simulink model "sim_generate_data"  (R2020b)
settings: Solver=FixedStepAuto  StartTime=0.0  StopTime=tsim  FixedStep=dt  RelTol=1e-3
undefined symbols (not defined in the file): A, B, C, dt, Fdiff_lin, Fsum_lin, K, Lobs, NOISE, noise_bound_data, t_disturb, u_disturb, x0
settings Model: Creator=Fabian  LastModifiedBy=Fabian

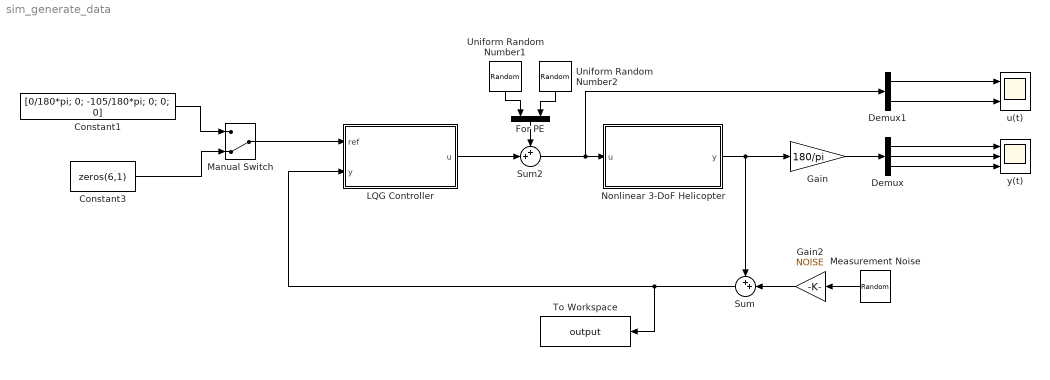
== system sim_generate_data ==
  Constant1 : Constant  Value=[0/180*pi; 0; -105/180*pi; 0; 0; 0]
  Constant3 : Constant  Value=zeros(6,1)
  Demux : Demux  Outputs=3
  Demux1 : Demux  Outputs=2
  For PE : Mux  Inputs=2
  Gain : Gain  Gain=180/pi
  Gain2 : Gain  Gain=NOISE
  LQG Controller : Subsystem
  Manual Switch : ManualSwitch  CurrentSetting=0
  Measurement Noise : UniformRandomNumber  Minimum=-noise_bound_data  Maximum=noise_bound_data  Seed=[0;1;2]  SampleTime=dt
  Nonlinear 3-DoF Helicopter : Subsystem
  Sum : Sum  Inputs=++|
  Sum2 : Sum  Inputs=++|
  To Workspace : ToWorkspace  VariableName=output  SaveFormat=Timeseries  SampleTime=-1
  Uniform Random Number1 : UniformRandomNumber  Minimum=-u_disturb  Maximum=u_disturb  SampleTime=t_disturb  VectorParams1D=off
  Uniform Random Number2 : UniformRandomNumber  Minimum=-u_disturb  Maximum=u_disturb  Seed=1  SampleTime=t_disturb  VectorParams1D=off
  u(t) : Scope  NumInputPorts=2
  y(t) : Scope  NumInputPorts=3
  wires:
  Sum/1 -> LQG Controller/2(y), To Workspace/1
  Uniform Random Number1/1 -> For PE/1
  Uniform Random Number2/1 -> For PE/2
  For PE/1 -> Sum2/1
  Nonlinear 3-DoF Helicopter/1(y) -> Gain/1, Sum/1
  Demux/3 -> y(t)/3
  Sum2/1 -> Nonlinear 3-DoF Helicopter/1(u), Demux1/1
  Demux/1 -> y(t)/1
  Demux/2 -> y(t)/2
  Demux1/1 -> u(t)/1
  Gain/1 -> Demux/1
  Demux1/2 -> u(t)/2
  Measurement Noise/1 -> Gain2/1
  Gain2/1 -> Sum/2
  Constant1/1 -> Manual Switch/1
  Constant3/1 -> Manual Switch/2
  Manual Switch/1 -> LQG Controller/1(ref)
  LQG Controller/1(u) -> Sum2/2

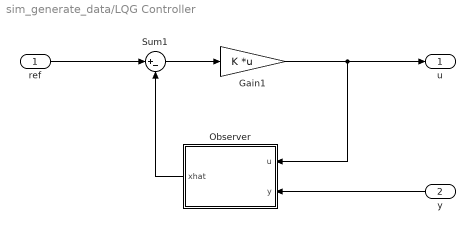
== system sim_generate_data/LQG Controller ==
  ref : Inport
  y : Inport  Port=2
  Gain1 : Gain  Gain=K  Multiplication=Matrix(K*u)
  Observer : Subsystem
  Sum1 : Sum  Inputs=|+-
  u : Outport
  wires:
  Observer/1(xhat) -> Sum1/2
  Gain1/1 -> Observer/1(u), u/1
  Sum1/1 -> Gain1/1
  ref/1 -> Sum1/1
  y/1 -> Observer/2(y)

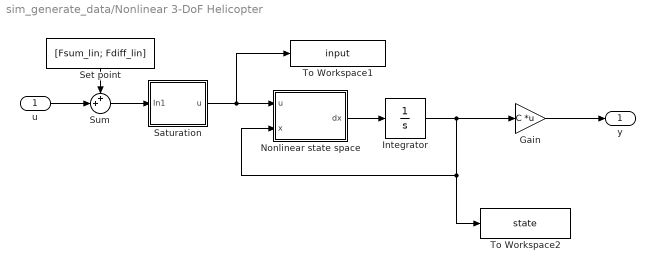
== system sim_generate_data/Nonlinear 3-DoF Helicopter ==
  u : Inport
  Gain : Gain  Gain=C  Multiplication=Matrix(K*u)
  Integrator : Integrator  InitialCondition=x0
  Nonlinear state space : MATLAB Function  TreatAsAtomicUnit=on
  Saturation : Subsystem
  Set point : Constant  Value=[Fsum_lin; Fdiff_lin]
  Sum : Sum  Inputs=++|
  To Workspace1 : ToWorkspace  VariableName=input  SaveFormat=Timeseries  SampleTime=-1
  To Workspace2 : ToWorkspace  VariableName=state  SaveFormat=Timeseries  SampleTime=-1
  y : Outport
  wires:
  Nonlinear state space/1(dx) -> Integrator/1
  Gain/1 -> y/1
  Integrator/1 -> To Workspace2/1, Nonlinear state space/2(x), Gain/1
  Set point/1 -> Sum/1
  u/1 -> Sum/2
  Sum/1 -> Saturation/1(In1)
  Saturation/1(u) -> Nonlinear state space/1(u), To Workspace1/1

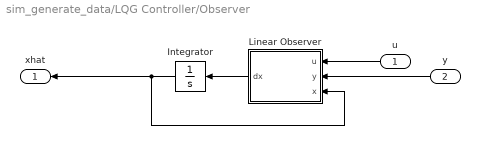
== system sim_generate_data/LQG Controller/Observer ==
  u : Inport
  y : Inport  Port=2
  Integrator : Integrator  InitialCondition=x0
  Linear Observer : MATLAB Function  TreatAsAtomicUnit=on
  xhat : Outport
  wires:
  u/1 -> Linear Observer/1(u)
  Integrator/1 -> Linear Observer/3(x), xhat/1
  Linear Observer/1(dx) -> Integrator/1
  y/1 -> Linear Observer/2(y)

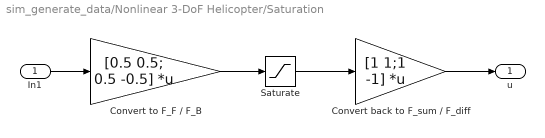
== system sim_generate_data/Nonlinear 3-DoF Helicopter/Saturation ==
  In1 : Inport
  Convert back to F_sum / F_diff : Gain  Gain=[1 1;1 -1]  Multiplication=Matrix(K*u)
  Convert to F_F / F_B : Gain  Gain=[0.5 0.5; 0.5 -0.5]  Multiplication=Matrix(K*u)
  Saturate : Saturate  UpperLimit=[0.98; 0.98]  LowerLimit=[0; 0]
  u : Outport
  wires:
  Convert back to F_sum / F_diff/1 -> u/1
  In1/1 -> Convert to F_F / F_B/1
  Convert to F_F / F_B/1 -> Saturate/1
  Saturate/1 -> Convert back to F_sum / F_diff/1

== matlab function sim_generate_data/LQG Controller/Observer/Linear Observer ==
  data: u input; y input; x input; dx output; A parameter; B parameter; Lobs parameter; C parameter
function dx = fcn(u,y,x, A, B, Lobs, C)

   dx = A*x + B*u + Lobs*(y - C*x); 

end

== matlab function sim_generate_data/Nonlinear 3-DoF Helicopter/Nonlinear state space ==
  data: u input; x input; dx output
function dx = fcn(u,x)

    m_H = 1.322;
    m_A = 2.638;

    Jxx = 1.1455;
    Jyy = 1.1184;
    Jzz = 0.032;

    r = 0.1775;

    rHx = -0.089;
    rHz = 0.655;
    rAHx = -0.034;
    rAHz = 0.0193;

    g = 9.81;
    
    dalph = x(2);
    bet = x(3);
    dbet = x(4);
    gam = x(5);
    dgam = x(6);
    
    Fsum = u(1);
    Fdiff = u(2);
    
    dx = [dalph;...
     1/Jxx * Fsum*sin(gam) * (rHx*sin(bet) - rHz*cos(bet));...
     dbet;...
     1/Jyy * (-(m_A+m_H)*g *(rAHz*cos(bet) - rAHx*sin(bet)) + Fsum * rHz*cos(gam));...
     dgam;...
     -1/Jzz * r * Fdiff];

end
